simulink model "lab2_task4"  (R2023a)
settings: Solver=VariableStepAuto  StartTime=0.0  StopTime=10.0  RelTol=1e-3
settings Model: Creator=MUHAMMAD SADEEQ  LastModifiedBy=MUHAMMAD SADEEQ

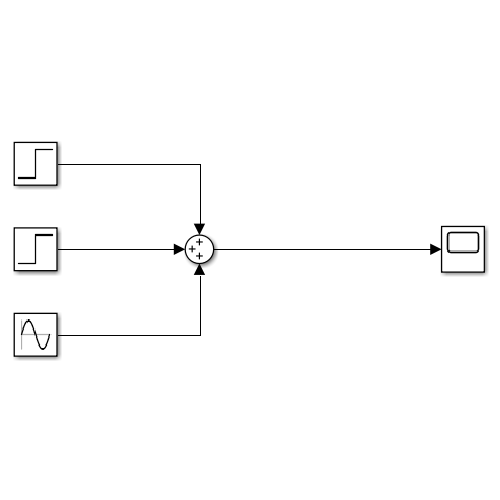
[thumbnail: Simulink's stored preview of the top-level diagram]
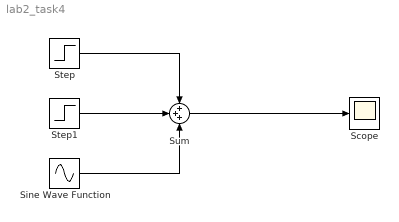
== system lab2_task4 ==
  Scope : Scope
  Sine Wave Function : Sin  Frequency=2*pi  SampleTime=0
  Step : Step  SampleTime=0
  Step1 : Step  Time=5  After=2  SampleTime=0
  Sum : Sum  Inputs=+++
  wires:
  Step/1 -> Sum/1
  Step1/1 -> Sum/2
  Sine Wave Function/1 -> Sum/3
  Sum/1 -> Scope/1
